simulink model "untitled"  (R2022b)
settings: Solver=FixedStepAuto  StartTime=0.0  StopTime=0.007*2500  FixedStep=0.007  RelTol=1e-3
values from neighbouring files (symbols this model uses):
  K = lqr(sys_ss,Q,R)    [main.m]
  Rw = 0.0216    [main.m]
undefined symbols (not defined in the file or in its folder): DiscIntNeverNeededParam, TS
libraries: RASPlib x3, simulink x3, MinSegLibrary_M1V4 x2, arduinolib x2
settings Model: ExtModeTrigDuration=2  Creator=Zuhair  LastModifiedBy=Zuhair
settings OptimizationCC: EnhancedBackFolding=on  PassReuseOutputArgsAs=Individual arguments  ZeroExternalMemoryAtStartup=off  ZeroInternalMemoryAtStartup=off  MaxStackSize=64  OptimizeBlockOrder=speed  DifferentSizesBufferReuse=on  OptimizationCustomize=off  EfficientTunableParamExpr=on
settings DebuggingCC: ParameterTunabilityLossMsg=error
settings HardwareCC: ProdBitPerInt=16  ProdBitPerPointer=16  ProdBitPerSizeT=16  ProdBitPerPtrDiffT=16  ProdLargestAtomicFloat=None  ProdWordSize=8  ProdHWDeviceType=Atmel->AVR  UseEmbeddedCoderFeatures=off  UseSimulinkCoderFeatures=off
settings SFSimCC: MATLABDynamicMemAlloc=off
settings RTWCC: Description=Embedded Coder  SystemTargetFile=ert.tlc  HardwareBoard=Arduino Mega 2560  TLCOptions=-aInlineSetEventsForThisBaseRateFcn=TLC_FALSE -aSuppressMultiTaskScheduler=TLC_FALSE -aRateBasedStepFcn=1  TemplateMakefile=ert_default_tmf  Toolchain=Arduino AVR
settings CodeAppCC: ForceParamTrailComments=on  IgnoreCustomStorageClasses=off  OperatorAnnotations=on  SimulinkDataObjDesc=on  SFDataObjDesc=on  MangleLength=10  InsertBlockDesc=on
settings ERTTargetCC: SupportContinuousTime=on  SupportNonInlinedSFcns=on  SupportVariableSizeSignals=on  ExtModeTransport=3  ExtModeStaticAlloc=on  ExtModeAutomaticAllocSize=off  ExtModeStaticAllocSize=2048  ExtModeMexFile=ext_xcp  ExtModeIntrfLevel=Level2 - Open

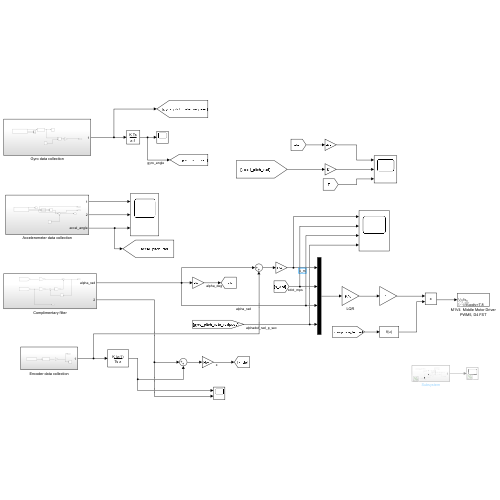
[thumbnail: Simulink's stored preview of the top-level diagram]
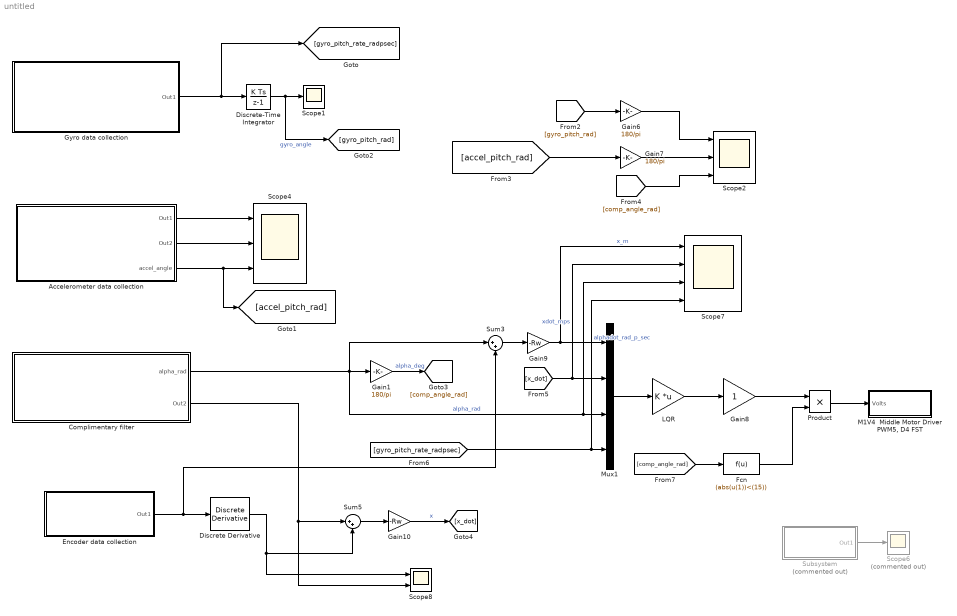
== system untitled ==
  Accelerometer data collection : Subsystem
  Complimentary filter : Subsystem
  Discrete Derivative : simulink/Discrete/Discrete Derivative  gainval=1.0  ICPrevScaledInput=0.0  OutMin=[]  OutMax=[]  OutDataType=fixdt(1, 16)  OutScaling=2^-10  DoSatur=off
  Discrete-Time Integrator : DiscreteIntegrator  SampleTime=-1  ICPrevOutput=DiscIntNeverNeededParam  ICPrevScaledInput=DiscIntNeverNeededParam
  Encoder data collection : Subsystem
  Fcn : Fcn  Expr=(abs(u(1))<(15))
  Gain1 : Gain  Gain=180/pi
  Gain10 : Gain  Gain=-Rw
  Gain6 : Gain  Gain=180/pi
  Gain7 : Gain  Gain=180/pi
  Gain8 : Gain
  Gain9 : Gain  Gain=-Rw
  Gyro data collection : Subsystem
  LQR : Gain  Gain=K  Multiplication=Matrix(K*u)
  "M1V4  Middle Motor Driver PWM5, D4 FST" : Subsystem  AncestorBlock="MinSegLibrary_M1V4/M1V4  Middle Motor Driver PWM5, D4 FST"  mask(Motor Driver){Vsupply=7.8}
      mask prompts: Vsupply "Driver Supply Voltage"
      mask help:
      | Use a single PWM and a single Digtial out to control the magnitude and direction of a motor
      |
      | Specify driver supply voltage (~3.25 for USB with SN754410)
      |
      | Driver supply voltage can be measured direcly by turning the motor fully on (100% duty cycle) and measuring the voltage across the motor leads.  This is the maximum voltage available to the motor and is used to scale from volts to PWM value 0-255.
      |
      | Note this value must be changed if the supply voltage to the driver is changed, for example, by using batteries.
      |
      | Vsupply is the maximum voltage your system is capable of supplying to system given the power supply. It needs to be measured depending on the power supply.
      settings: LibrarySourceBlock=|
      | MinSegLibrary_M1V4/M1V4  Middle Motor Driver
      | PWM5, D4 FST
      mask Display:
      | port_label('input',1,'Volts')
      | text(15,5,['Vsupply=' num2str(Vsupply)])
  Mux1 : Mux
  Product : Product
  Scope1 : Scope
  Scope2 : Scope  NumInputPorts=3
  Scope4 : Scope  NumInputPorts=3
  Scope6 : Scope  Commented=on
  Scope7 : Scope  NumInputPorts=4
  Scope8 : Scope  NumInputPorts=2
  Subsystem : Subsystem  Commented=on
  Sum3 : Sum  Inputs=|++
  Sum5 : Sum  Inputs=|++
  wires:
  Discrete-Time Integrator/1 -> [gyro_pitch_rad], Scope1/1  "gyro_angle"
  [accel_pitch_rad] -> Gain7/1
  [comp_angle_rad] -> Scope2/3
  [gyro_pitch_rad] -> Gain6/1
  Gain6/1 -> Scope2/1
  Gain7/1 -> Scope2/2
  LQR/1 -> Gain8/1
  Mux1/1 -> LQR/1
  Gain9/1 -> Scope7/1, Mux1/1  "x_m"
  [x_dot] -> Mux1/2, Scope7/2  "xdot_mps"
  Gain1/1 -> [comp_angle_rad]  "alpha_deg"
  Sum3/1 -> Gain9/1
  Discrete Derivative/1 -> Scope8/1, Sum5/2
  Sum5/1 -> Gain10/1
  Gain10/1 -> [x_dot]  "x"
  [comp_angle_rad] -> Fcn/1
  Gain8/1 -> Product/1
  Fcn/1 -> Product/2
  Subsystem/1(Out1) -> Scope6/1
  Product/1 -> "M1V4  Middle Motor Driver PWM5, D4 FST"/1(Volts)
  [gyro_pitch_rate_radpsec] -> Scope7/4, Mux1/4  "alphadot_rad_p_sec"
  Gyro data collection/1(Out1) -> [gyro_pitch_rate_radpsec], Discrete-Time Integrator/1
  Accelerometer data collection/3(accel_angle) -> [accel_pitch_rad], Scope4/3
  Accelerometer data collection/1(Out1) -> Scope4/1
  Accelerometer data collection/2(Out2) -> Scope4/2
  Encoder data collection/1(Out1) -> Sum3/2, Discrete Derivative/1
  Complimentary filter/1(alpha_rad) -> Mux1/3, Scope7/3, Gain1/1, Sum3/1  "alpha_rad"
  Complimentary filter/2(Out2) -> Scope8/2, Sum5/1

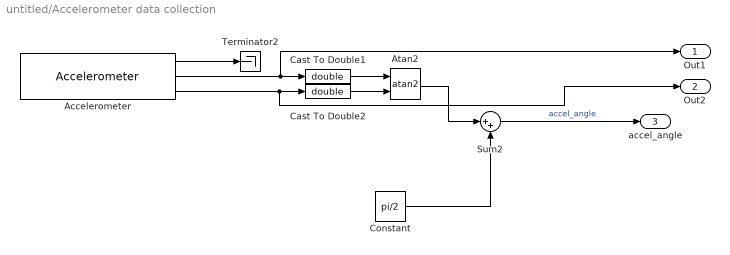
== system untitled/Accelerometer data collection ==
  Accelerometer : RASPlib/Accelerometer  SimulateUsing=Code generation
      settings: SourceProductName=Rensselaer Arduino Support Package
  Atan2 : Trigonometry  Operator=atan2
  Cast To Double1 : DataTypeConversion  OutDataTypeStr=double  SaturateOnIntegerOverflow=off  RndMeth=Floor
  Cast To Double2 : DataTypeConversion  OutDataTypeStr=double  SaturateOnIntegerOverflow=off  RndMeth=Floor
  Constant : Constant  Value=pi/2
  Sum2 : Sum  Inputs=|++
  Terminator2 : Terminator
  Out1 : Outport
  Out2 : Outport  Port=2
  accel_angle : Outport  Port=3
  wires:
  Sum2/1 -> accel_angle/1  "accel_angle"
  Accelerometer/3 -> Out2/1, Cast To Double2/1
  Cast To Double1/1 -> Atan2/1
  Accelerometer/2 -> Out1/1, Cast To Double1/1
  Cast To Double2/1 -> Atan2/2
  Atan2/1 -> Sum2/1
  Accelerometer/1 -> Terminator2/1
  Constant/1 -> Sum2/2

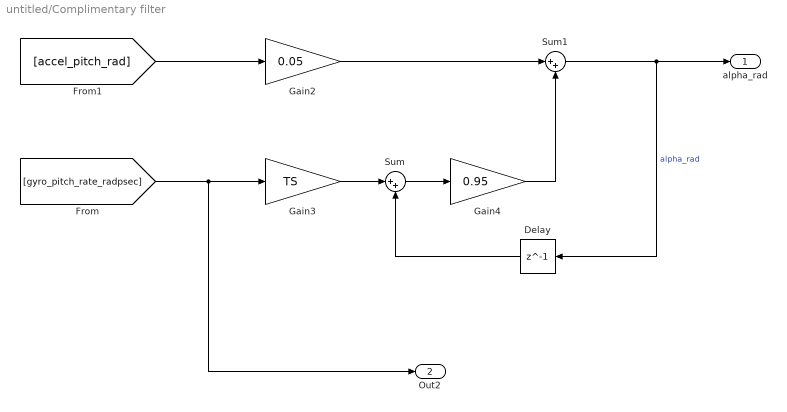
== system untitled/Complimentary filter ==
  Delay : Delay  DelayLength=1  SampleTime=0.007
  Gain2 : Gain  Gain=0.05
  Gain3 : Gain  Gain=TS
  Gain4 : Gain  Gain=0.95
  Sum : Sum  Inputs=|++
  Sum1 : Sum  Inputs=|++
  alpha_rad : Outport
  Out2 : Outport  Port=2
  wires:
  [accel_pitch_rad] -> Gain2/1
  [gyro_pitch_rate_radpsec] -> Out2/1, Gain3/1
  Sum1/1 -> alpha_rad/1, Delay/1  "alpha_rad"
  Sum/1 -> Gain4/1
  Gain3/1 -> Sum/1
  Delay/1 -> Sum/2
  Gain2/1 -> Sum1/1
  Gain4/1 -> Sum1/2

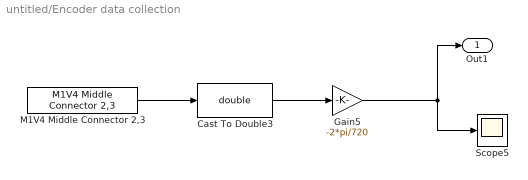
== system untitled/Encoder data collection ==
  Cast To Double3 : DataTypeConversion  OutDataTypeStr=double  SaturateOnIntegerOverflow=off  RndMeth=Floor
  Gain5 : Gain  Gain=-2*pi/720
  M1V4 Middle Connector 2,3 : MinSegLibrary_M1V4/M1V4 Middle Connector 2,3  Encoder=0  PinA=3  PinB=2
      settings: SourceProductName=Rensselaer Arduino Support Package
  Scope5 : Scope
  Out1 : Outport
  wires:
  Cast To Double3/1 -> Gain5/1
  Gain5/1 -> Out1/1, Scope5/1
  M1V4 Middle Connector 2,3/1 -> Cast To Double3/1

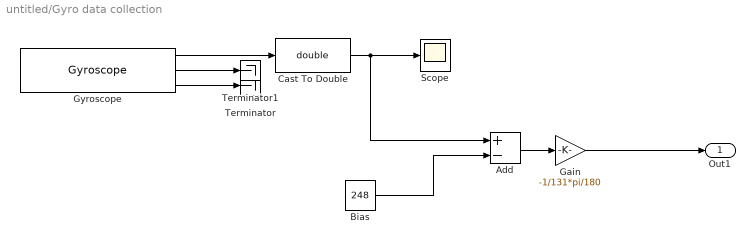
== system untitled/Gyro data collection ==
  Add : Sum  Inputs=+-
  Bias : Constant  Value=248
  Cast To Double : DataTypeConversion  OutDataTypeStr=double  SaturateOnIntegerOverflow=off  RndMeth=Floor
  Gain : Gain  Gain=-1/131*pi/180
  Gyroscope : RASPlib/Gyroscope  DLPFmode=0
      settings: SourceProductName=Rensselaer Arduino Support Package
  Scope : Scope
  Terminator : Terminator
  Terminator1 : Terminator
  Out1 : Outport
  wires:
  Cast To Double/1 -> Add/1, Scope/1
  Gain/1 -> Out1/1
  Add/1 -> Gain/1
  Gyroscope/3 -> Terminator/1
  Gyroscope/2 -> Terminator1/1
  Bias/1 -> Add/2
  Gyroscope/1 -> Cast To Double/1

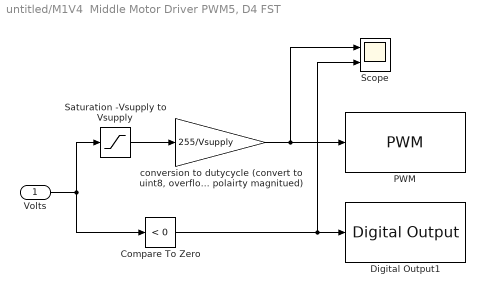
== system untitled/M1V4  Middle Motor Driver PWM5, D4 FST ==
  Volts : Inport
  Compare To Zero : simulink/Logic and Bit Operations/Compare To Zero  relop=<  OutDataTypeStr=boolean
  Digital Output1 : arduinolib/Digital Output  pinNumber=4  Direction=output  blockPlatform=arduino
  PWM : arduinolib/PWM  pinNumber=5  frequencyType=Default  desiredFrequency=490.2  achievableFrequency=490.2
  Saturation -Vsupply to Vsupply : Saturate  UpperLimit=Vsupply  LowerLimit=-Vsupply  OutDataTypeStr=single
  Scope : Scope  NumInputPorts=2
  "conversion to dutycycle (convert to uint8, overflow will provide reverse polairty magnitued)" : Gain  Gain=255/Vsupply  OutDataTypeStr=uint8
  wires:
  Compare To Zero/1 -> Scope/2, Digital Output1/1
  Saturation -Vsupply to Vsupply/1 -> "conversion to dutycycle (convert to uint8, overflow will provide reverse polairty magnitued)"/1
  Volts/1 -> Saturation -Vsupply to Vsupply/1, Compare To Zero/1
  "conversion to dutycycle (convert to uint8, overflow will provide reverse polairty magnitued)"/1 -> PWM/1, Scope/1

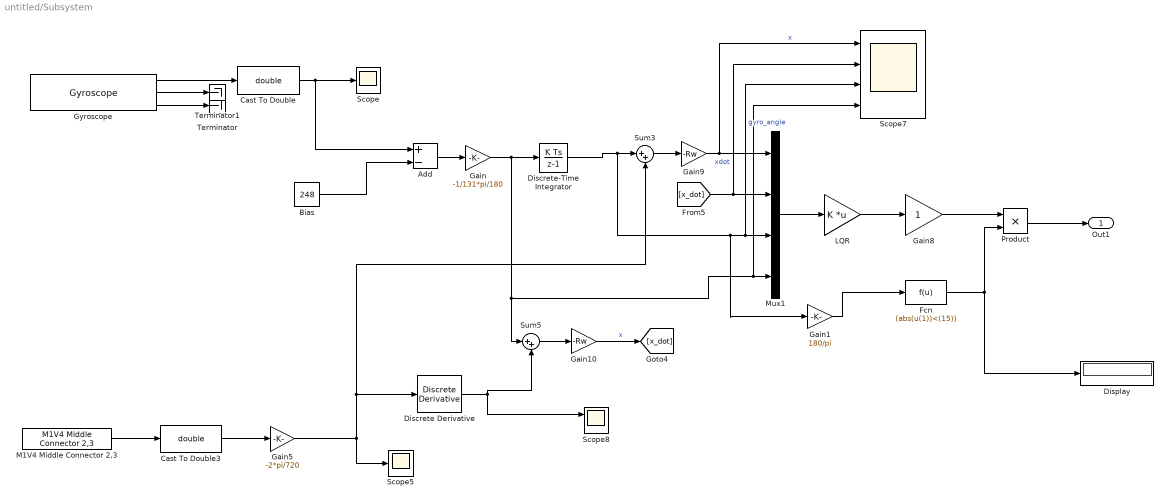
== system untitled/Subsystem ==
  Add : Sum  Inputs=+-
  Bias : Constant  Value=248
  Cast To Double : DataTypeConversion  OutDataTypeStr=double  SaturateOnIntegerOverflow=off  RndMeth=Floor
  Cast To Double3 : DataTypeConversion  OutDataTypeStr=double  SaturateOnIntegerOverflow=off  RndMeth=Floor
  Discrete Derivative : simulink/Discrete/Discrete Derivative  gainval=1.0  ICPrevScaledInput=0.0  OutMin=[]  OutMax=[]  OutDataType=fixdt(1, 16)  OutScaling=2^-10  DoSatur=off
  Discrete-Time Integrator : DiscreteIntegrator  SampleTime=-1  ICPrevOutput=DiscIntNeverNeededParam  ICPrevScaledInput=DiscIntNeverNeededParam
  Display : Display
  Fcn : Fcn  Expr=(abs(u(1))<(15))
  Gain : Gain  Gain=-1/131*pi/180
  Gain1 : Gain  Gain=180/pi
  Gain10 : Gain  Gain=-Rw
  Gain5 : Gain  Gain=-2*pi/720
  Gain8 : Gain
  Gain9 : Gain  Gain=-Rw
  Gyroscope : RASPlib/Gyroscope  DLPFmode=5
      settings: SourceProductName=Rensselaer Arduino Support Package
  LQR : Gain  Gain=K  Multiplication=Matrix(K*u)
  M1V4 Middle Connector 2,3 : MinSegLibrary_M1V4/M1V4 Middle Connector 2,3  Encoder=0  PinA=3  PinB=2
      settings: SourceProductName=Rensselaer Arduino Support Package
  Mux1 : Mux
  Product : Product
  Scope : Scope
  Scope5 : Scope
  Scope7 : Scope  NumInputPorts=4
  Scope8 : Scope  NumInputPorts=2
  Sum3 : Sum  Inputs=|++
  Sum5 : Sum  Inputs=|++
  Terminator : Terminator
  Terminator1 : Terminator
  Out1 : Outport
  wires:
  Product/1 -> Out1/1
  Fcn/1 -> Product/2, Display/1
  Gain8/1 -> Product/1
  Sum5/1 -> Gain10/1
  Gain10/1 -> [x_dot]  "x"
  Cast To Double3/1 -> Gain5/1
  Sum3/1 -> Gain9/1
  LQR/1 -> Gain8/1
  M1V4 Middle Connector 2,3/1 -> Cast To Double3/1
  Gain5/1 -> Scope5/1, Sum3/2, Discrete Derivative/1
  Gain9/1 -> Scope7/1, Mux1/1  "x"
  [x_dot] -> Mux1/2, Scope7/2  "xdot"
  Mux1/1 -> LQR/1
  Gyroscope/2 -> Terminator1/1
  Gyroscope/1 -> Cast To Double/1
  Cast To Double/1 -> Add/1, Scope/1
  Gain/1 -> Sum5/1, Scope7/4, Mux1/4, Discrete-Time Integrator/1
  Add/1 -> Gain/1
  Bias/1 -> Add/2
  Discrete-Time Integrator/1 -> Gain1/1, Scope7/3, Mux1/3, Sum3/1  "gyro_angle"
  Gyroscope/3 -> Terminator/1
  Discrete Derivative/1 -> Sum5/2, Scope8/1
  Gain1/1 -> Fcn/1
